simulink model "Project2"  (R2015a)
settings: Solver=ode45  StartTime=0.0  StopTime=10000  RelTol=1e-3
PreLoadFcn:
  | Init
InitFcn:
  | Init
values from neighbouring files (symbols this model uses):
  a = 5    [Init.m]
  b = 10    [Init.m]
  PACCPrecision = 32    [Init.m]
  seed = [1,2,3,4,5,6]    [Init.m]
undefined symbols (not defined in the file or in its folder): c
libraries: xbsIndex_r4 x91, xrbsComm_r4 x1
(part 2 of 2)

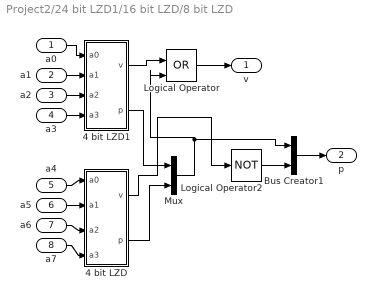
== system Project2/24 bit LZD1/16 bit LZD/8 bit LZD ==
  a0 : Inport
  a1 : Inport  Port=2
  a2 : Inport  Port=3
  a3 : Inport  Port=4
  a4 : Inport  Port=5
  a5 : Inport  Port=6
  a6 : Inport  Port=7
  a7 : Inport  Port=8
  4 bit LZD : Subsystem
  4 bit LZD1 : Subsystem
  Bus Creator1 : BusCreator  Inputs=2
  Logical Operator : Logic  Operator=OR  IconShape=distinctive  AllPortsSameDT=off  OutDataTypeStr=boolean
  Logical Operator2 : Logic  Operator=NOT  IconShape=distinctive  AllPortsSameDT=off  OutDataTypeStr=boolean
  Mux : Mux  Inputs=2
  v : Outport
  p : Outport  Port=2
  wires:
  a2/1 -> 4 bit LZD1/3(a2)
  a6/1 -> 4 bit LZD/3(a2)
  a7/1 -> 4 bit LZD/4(a3)
  a3/1 -> 4 bit LZD1/4(a3)
  a0/1 -> 4 bit LZD1/1(a0)
  a1/1 -> 4 bit LZD1/2(a1)
  a5/1 -> 4 bit LZD/2(a1)
  a4/1 -> 4 bit LZD/1(a0)
  Logical Operator/1 -> v/1
  Logical Operator2/1 -> Bus Creator1/2
  4 bit LZD1/1(v) -> Logical Operator/1
  Mux/1 -> Logical Operator/2, Bus Creator1/1
  4 bit LZD/2(p) -> Mux/2
  Bus Creator1/1 -> p/1
  4 bit LZD/1(v) -> Logical Operator2/1
  4 bit LZD1/2(p) -> Mux/1

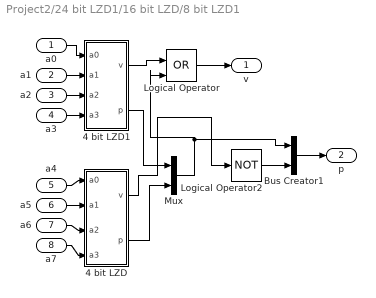
== system Project2/24 bit LZD1/16 bit LZD/8 bit LZD1 ==
  a0 : Inport
  a1 : Inport  Port=2
  a2 : Inport  Port=3
  a3 : Inport  Port=4
  a4 : Inport  Port=5
  a5 : Inport  Port=6
  a6 : Inport  Port=7
  a7 : Inport  Port=8
  4 bit LZD : Subsystem
  4 bit LZD1 : Subsystem
  Bus Creator1 : BusCreator  Inputs=2
  Logical Operator : Logic  Operator=OR  IconShape=distinctive  AllPortsSameDT=off  OutDataTypeStr=boolean
  Logical Operator2 : Logic  Operator=NOT  IconShape=distinctive  AllPortsSameDT=off  OutDataTypeStr=boolean
  Mux : Mux  Inputs=2
  v : Outport
  p : Outport  Port=2
  wires:
  a2/1 -> 4 bit LZD1/3(a2)
  a6/1 -> 4 bit LZD/3(a2)
  a7/1 -> 4 bit LZD/4(a3)
  a3/1 -> 4 bit LZD1/4(a3)
  a0/1 -> 4 bit LZD1/1(a0)
  a1/1 -> 4 bit LZD1/2(a1)
  a5/1 -> 4 bit LZD/2(a1)
  a4/1 -> 4 bit LZD/1(a0)
  Logical Operator/1 -> v/1
  Logical Operator2/1 -> Bus Creator1/2
  4 bit LZD1/1(v) -> Logical Operator/1
  Mux/1 -> Logical Operator/2, Bus Creator1/1
  4 bit LZD/2(p) -> Mux/2
  Bus Creator1/1 -> p/1
  4 bit LZD/1(v) -> Logical Operator2/1
  4 bit LZD1/2(p) -> Mux/1

== system Project2/24 bit LZD1/8 bit LZD/4 bit LZD ==
  a0 : Inport
  a1 : Inport  Port=2
  a2 : Inport  Port=3
  a3 : Inport  Port=4
  2 bit LZD : Subsystem
  2 bit LZD1 : Subsystem
  Bus Creator1 : BusCreator  Inputs=2
  Logical Operator : Logic  Operator=OR  IconShape=distinctive  AllPortsSameDT=off  OutDataTypeStr=boolean
  Logical Operator2 : Logic  Operator=NOT  IconShape=distinctive  AllPortsSameDT=off  OutDataTypeStr=boolean
  Mux : Mux  Inputs=2
  v : Outport
  p : Outport  Port=2
  wires:
  2 bit LZD/1(v) -> Logical Operator2/1
  2 bit LZD1/2(p) -> Mux/1
  2 bit LZD/2(p) -> Mux/2
  Bus Creator1/1 -> p/1
  a0/1 -> 2 bit LZD1/1(a0)
  a2/1 -> 2 bit LZD/1(a0)
  a1/1 -> 2 bit LZD1/2(a1)
  a3/1 -> 2 bit LZD/2(a1)
  Logical Operator/1 -> v/1
  2 bit LZD1/1(v) -> Logical Operator/1
  Logical Operator2/1 -> Bus Creator1/2
  Mux/1 -> Logical Operator/2, Bus Creator1/1

== system Project2/24 bit LZD1/8 bit LZD/4 bit LZD1 ==
  a0 : Inport
  a1 : Inport  Port=2
  a2 : Inport  Port=3
  a3 : Inport  Port=4
  2 bit LZD : Subsystem
  2 bit LZD1 : Subsystem
  Bus Creator1 : BusCreator  Inputs=2
  Logical Operator : Logic  Operator=OR  IconShape=distinctive  AllPortsSameDT=off  OutDataTypeStr=boolean
  Logical Operator2 : Logic  Operator=NOT  IconShape=distinctive  AllPortsSameDT=off  OutDataTypeStr=boolean
  Mux : Mux  Inputs=2
  v : Outport
  p : Outport  Port=2
  wires:
  2 bit LZD/1(v) -> Logical Operator2/1
  2 bit LZD1/2(p) -> Mux/1
  2 bit LZD/2(p) -> Mux/2
  Bus Creator1/1 -> p/1
  a0/1 -> 2 bit LZD1/1(a0)
  a2/1 -> 2 bit LZD/1(a0)
  a1/1 -> 2 bit LZD1/2(a1)
  a3/1 -> 2 bit LZD/2(a1)
  Logical Operator/1 -> v/1
  2 bit LZD1/1(v) -> Logical Operator/1
  Logical Operator2/1 -> Bus Creator1/2
  Mux/1 -> Logical Operator/2, Bus Creator1/1

== system Project2/24 bit LZD/16 bit LZD/8 bit LZD/4 bit LZD ==
  a0 : Inport
  a1 : Inport  Port=2
  a2 : Inport  Port=3
  a3 : Inport  Port=4
  2 bit LZD : Subsystem
  2 bit LZD1 : Subsystem
  Bus Creator1 : BusCreator  Inputs=2
  Logical Operator : Logic  Operator=OR  IconShape=distinctive  AllPortsSameDT=off  OutDataTypeStr=boolean
  Logical Operator2 : Logic  Operator=NOT  IconShape=distinctive  AllPortsSameDT=off  OutDataTypeStr=boolean
  Mux : Mux  Inputs=2
  v : Outport
  p : Outport  Port=2
  wires:
  2 bit LZD/1(v) -> Logical Operator2/1
  2 bit LZD1/2(p) -> Mux/1
  2 bit LZD/2(p) -> Mux/2
  Bus Creator1/1 -> p/1
  a0/1 -> 2 bit LZD1/1(a0)
  a2/1 -> 2 bit LZD/1(a0)
  a1/1 -> 2 bit LZD1/2(a1)
  a3/1 -> 2 bit LZD/2(a1)
  Logical Operator/1 -> v/1
  2 bit LZD1/1(v) -> Logical Operator/1
  Logical Operator2/1 -> Bus Creator1/2
  Mux/1 -> Logical Operator/2, Bus Creator1/1

== system Project2/24 bit LZD/16 bit LZD/8 bit LZD/4 bit LZD1 ==
  a0 : Inport
  a1 : Inport  Port=2
  a2 : Inport  Port=3
  a3 : Inport  Port=4
  2 bit LZD : Subsystem
  2 bit LZD1 : Subsystem
  Bus Creator1 : BusCreator  Inputs=2
  Logical Operator : Logic  Operator=OR  IconShape=distinctive  AllPortsSameDT=off  OutDataTypeStr=boolean
  Logical Operator2 : Logic  Operator=NOT  IconShape=distinctive  AllPortsSameDT=off  OutDataTypeStr=boolean
  Mux : Mux  Inputs=2
  v : Outport
  p : Outport  Port=2
  wires:
  2 bit LZD/1(v) -> Logical Operator2/1
  2 bit LZD1/2(p) -> Mux/1
  2 bit LZD/2(p) -> Mux/2
  Bus Creator1/1 -> p/1
  a0/1 -> 2 bit LZD1/1(a0)
  a2/1 -> 2 bit LZD/1(a0)
  a1/1 -> 2 bit LZD1/2(a1)
  a3/1 -> 2 bit LZD/2(a1)
  Logical Operator/1 -> v/1
  2 bit LZD1/1(v) -> Logical Operator/1
  Logical Operator2/1 -> Bus Creator1/2
  Mux/1 -> Logical Operator/2, Bus Creator1/1

== system Project2/24 bit LZD/16 bit LZD/8 bit LZD1/4 bit LZD ==
  a0 : Inport
  a1 : Inport  Port=2
  a2 : Inport  Port=3
  a3 : Inport  Port=4
  2 bit LZD : Subsystem
  2 bit LZD1 : Subsystem
  Bus Creator1 : BusCreator  Inputs=2
  Logical Operator : Logic  Operator=OR  IconShape=distinctive  AllPortsSameDT=off  OutDataTypeStr=boolean
  Logical Operator2 : Logic  Operator=NOT  IconShape=distinctive  AllPortsSameDT=off  OutDataTypeStr=boolean
  Mux : Mux  Inputs=2
  v : Outport
  p : Outport  Port=2
  wires:
  2 bit LZD/1(v) -> Logical Operator2/1
  2 bit LZD1/2(p) -> Mux/1
  2 bit LZD/2(p) -> Mux/2
  Bus Creator1/1 -> p/1
  a0/1 -> 2 bit LZD1/1(a0)
  a2/1 -> 2 bit LZD/1(a0)
  a1/1 -> 2 bit LZD1/2(a1)
  a3/1 -> 2 bit LZD/2(a1)
  Logical Operator/1 -> v/1
  2 bit LZD1/1(v) -> Logical Operator/1
  Logical Operator2/1 -> Bus Creator1/2
  Mux/1 -> Logical Operator/2, Bus Creator1/1

== system Project2/24 bit LZD/16 bit LZD/8 bit LZD1/4 bit LZD1 ==
  a0 : Inport
  a1 : Inport  Port=2
  a2 : Inport  Port=3
  a3 : Inport  Port=4
  2 bit LZD : Subsystem
  2 bit LZD1 : Subsystem
  Bus Creator1 : BusCreator  Inputs=2
  Logical Operator : Logic  Operator=OR  IconShape=distinctive  AllPortsSameDT=off  OutDataTypeStr=boolean
  Logical Operator2 : Logic  Operator=NOT  IconShape=distinctive  AllPortsSameDT=off  OutDataTypeStr=boolean
  Mux : Mux  Inputs=2
  v : Outport
  p : Outport  Port=2
  wires:
  2 bit LZD/1(v) -> Logical Operator2/1
  2 bit LZD1/2(p) -> Mux/1
  2 bit LZD/2(p) -> Mux/2
  Bus Creator1/1 -> p/1
  a0/1 -> 2 bit LZD1/1(a0)
  a2/1 -> 2 bit LZD/1(a0)
  a1/1 -> 2 bit LZD1/2(a1)
  a3/1 -> 2 bit LZD/2(a1)
  Logical Operator/1 -> v/1
  2 bit LZD1/1(v) -> Logical Operator/1
  Logical Operator2/1 -> Bus Creator1/2
  Mux/1 -> Logical Operator/2, Bus Creator1/1

== system Project2/24 bit LZD/8 bit LZD/4 bit LZD/2 bit LZD ==
  a0 : Inport
  a1 : Inport  Port=2
  Logical Operator : Logic  Operator=OR  IconShape=distinctive  AllPortsSameDT=off  OutDataTypeStr=boolean
  Logical Operator1 : Logic  IconShape=distinctive  AllPortsSameDT=off  OutDataTypeStr=boolean
  Logical Operator2 : Logic  Operator=NOT  IconShape=distinctive  AllPortsSameDT=off  OutDataTypeStr=boolean
  v : Outport
  p : Outport  Port=2
  wires:
  Logical Operator/1 -> v/1
  Logical Operator2/1 -> Logical Operator1/2
  a0/1 -> Logical Operator1/1, Logical Operator/1
  Logical Operator1/1 -> p/1
  a1/1 -> Logical Operator/2, Logical Operator2/1

== system Project2/24 bit LZD/8 bit LZD/4 bit LZD/2 bit LZD1 ==
  a0 : Inport
  a1 : Inport  Port=2
  Logical Operator : Logic  Operator=OR  IconShape=distinctive  AllPortsSameDT=off  OutDataTypeStr=boolean
  Logical Operator1 : Logic  IconShape=distinctive  AllPortsSameDT=off  OutDataTypeStr=boolean
  Logical Operator2 : Logic  Operator=NOT  IconShape=distinctive  AllPortsSameDT=off  OutDataTypeStr=boolean
  v : Outport
  p : Outport  Port=2
  wires:
  Logical Operator/1 -> v/1
  Logical Operator2/1 -> Logical Operator1/2
  a0/1 -> Logical Operator1/1, Logical Operator/1
  Logical Operator1/1 -> p/1
  a1/1 -> Logical Operator/2, Logical Operator2/1

== system Project2/24 bit LZD/8 bit LZD/4 bit LZD1/2 bit LZD ==
  a0 : Inport
  a1 : Inport  Port=2
  Logical Operator : Logic  Operator=OR  IconShape=distinctive  AllPortsSameDT=off  OutDataTypeStr=boolean
  Logical Operator1 : Logic  IconShape=distinctive  AllPortsSameDT=off  OutDataTypeStr=boolean
  Logical Operator2 : Logic  Operator=NOT  IconShape=distinctive  AllPortsSameDT=off  OutDataTypeStr=boolean
  v : Outport
  p : Outport  Port=2
  wires:
  Logical Operator/1 -> v/1
  Logical Operator2/1 -> Logical Operator1/2
  a0/1 -> Logical Operator1/1, Logical Operator/1
  Logical Operator1/1 -> p/1
  a1/1 -> Logical Operator/2, Logical Operator2/1

== system Project2/24 bit LZD/8 bit LZD/4 bit LZD1/2 bit LZD1 ==
  a0 : Inport
  a1 : Inport  Port=2
  Logical Operator : Logic  Operator=OR  IconShape=distinctive  AllPortsSameDT=off  OutDataTypeStr=boolean
  Logical Operator1 : Logic  IconShape=distinctive  AllPortsSameDT=off  OutDataTypeStr=boolean
  Logical Operator2 : Logic  Operator=NOT  IconShape=distinctive  AllPortsSameDT=off  OutDataTypeStr=boolean
  v : Outport
  p : Outport  Port=2
  wires:
  Logical Operator/1 -> v/1
  Logical Operator2/1 -> Logical Operator1/2
  a0/1 -> Logical Operator1/1, Logical Operator/1
  Logical Operator1/1 -> p/1
  a1/1 -> Logical Operator/2, Logical Operator2/1

== system Project2/24 bit LZD1/16 bit LZD/8 bit LZD/4 bit LZD ==
  a0 : Inport
  a1 : Inport  Port=2
  a2 : Inport  Port=3
  a3 : Inport  Port=4
  2 bit LZD : Subsystem
  2 bit LZD1 : Subsystem
  Bus Creator1 : BusCreator  Inputs=2
  Logical Operator : Logic  Operator=OR  IconShape=distinctive  AllPortsSameDT=off  OutDataTypeStr=boolean
  Logical Operator2 : Logic  Operator=NOT  IconShape=distinctive  AllPortsSameDT=off  OutDataTypeStr=boolean
  Mux : Mux  Inputs=2
  v : Outport
  p : Outport  Port=2
  wires:
  2 bit LZD/1(v) -> Logical Operator2/1
  2 bit LZD1/2(p) -> Mux/1
  2 bit LZD/2(p) -> Mux/2
  Bus Creator1/1 -> p/1
  a0/1 -> 2 bit LZD1/1(a0)
  a2/1 -> 2 bit LZD/1(a0)
  a1/1 -> 2 bit LZD1/2(a1)
  a3/1 -> 2 bit LZD/2(a1)
  Logical Operator/1 -> v/1
  2 bit LZD1/1(v) -> Logical Operator/1
  Logical Operator2/1 -> Bus Creator1/2
  Mux/1 -> Logical Operator/2, Bus Creator1/1

== system Project2/24 bit LZD1/16 bit LZD/8 bit LZD/4 bit LZD1 ==
  a0 : Inport
  a1 : Inport  Port=2
  a2 : Inport  Port=3
  a3 : Inport  Port=4
  2 bit LZD : Subsystem
  2 bit LZD1 : Subsystem
  Bus Creator1 : BusCreator  Inputs=2
  Logical Operator : Logic  Operator=OR  IconShape=distinctive  AllPortsSameDT=off  OutDataTypeStr=boolean
  Logical Operator2 : Logic  Operator=NOT  IconShape=distinctive  AllPortsSameDT=off  OutDataTypeStr=boolean
  Mux : Mux  Inputs=2
  v : Outport
  p : Outport  Port=2
  wires:
  2 bit LZD/1(v) -> Logical Operator2/1
  2 bit LZD1/2(p) -> Mux/1
  2 bit LZD/2(p) -> Mux/2
  Bus Creator1/1 -> p/1
  a0/1 -> 2 bit LZD1/1(a0)
  a2/1 -> 2 bit LZD/1(a0)
  a1/1 -> 2 bit LZD1/2(a1)
  a3/1 -> 2 bit LZD/2(a1)
  Logical Operator/1 -> v/1
  2 bit LZD1/1(v) -> Logical Operator/1
  Logical Operator2/1 -> Bus Creator1/2
  Mux/1 -> Logical Operator/2, Bus Creator1/1

== system Project2/24 bit LZD1/16 bit LZD/8 bit LZD1/4 bit LZD ==
  a0 : Inport
  a1 : Inport  Port=2
  a2 : Inport  Port=3
  a3 : Inport  Port=4
  2 bit LZD : Subsystem
  2 bit LZD1 : Subsystem
  Bus Creator1 : BusCreator  Inputs=2
  Logical Operator : Logic  Operator=OR  IconShape=distinctive  AllPortsSameDT=off  OutDataTypeStr=boolean
  Logical Operator2 : Logic  Operator=NOT  IconShape=distinctive  AllPortsSameDT=off  OutDataTypeStr=boolean
  Mux : Mux  Inputs=2
  v : Outport
  p : Outport  Port=2
  wires:
  2 bit LZD/1(v) -> Logical Operator2/1
  2 bit LZD1/2(p) -> Mux/1
  2 bit LZD/2(p) -> Mux/2
  Bus Creator1/1 -> p/1
  a0/1 -> 2 bit LZD1/1(a0)
  a2/1 -> 2 bit LZD/1(a0)
  a1/1 -> 2 bit LZD1/2(a1)
  a3/1 -> 2 bit LZD/2(a1)
  Logical Operator/1 -> v/1
  2 bit LZD1/1(v) -> Logical Operator/1
  Logical Operator2/1 -> Bus Creator1/2
  Mux/1 -> Logical Operator/2, Bus Creator1/1

== system Project2/24 bit LZD1/16 bit LZD/8 bit LZD1/4 bit LZD1 ==
  a0 : Inport
  a1 : Inport  Port=2
  a2 : Inport  Port=3
  a3 : Inport  Port=4
  2 bit LZD : Subsystem
  2 bit LZD1 : Subsystem
  Bus Creator1 : BusCreator  Inputs=2
  Logical Operator : Logic  Operator=OR  IconShape=distinctive  AllPortsSameDT=off  OutDataTypeStr=boolean
  Logical Operator2 : Logic  Operator=NOT  IconShape=distinctive  AllPortsSameDT=off  OutDataTypeStr=boolean
  Mux : Mux  Inputs=2
  v : Outport
  p : Outport  Port=2
  wires:
  2 bit LZD/1(v) -> Logical Operator2/1
  2 bit LZD1/2(p) -> Mux/1
  2 bit LZD/2(p) -> Mux/2
  Bus Creator1/1 -> p/1
  a0/1 -> 2 bit LZD1/1(a0)
  a2/1 -> 2 bit LZD/1(a0)
  a1/1 -> 2 bit LZD1/2(a1)
  a3/1 -> 2 bit LZD/2(a1)
  Logical Operator/1 -> v/1
  2 bit LZD1/1(v) -> Logical Operator/1
  Logical Operator2/1 -> Bus Creator1/2
  Mux/1 -> Logical Operator/2, Bus Creator1/1

== system Project2/24 bit LZD1/8 bit LZD/4 bit LZD/2 bit LZD ==
  a0 : Inport
  a1 : Inport  Port=2
  Logical Operator : Logic  Operator=OR  IconShape=distinctive  AllPortsSameDT=off  OutDataTypeStr=boolean
  Logical Operator1 : Logic  IconShape=distinctive  AllPortsSameDT=off  OutDataTypeStr=boolean
  Logical Operator2 : Logic  Operator=NOT  IconShape=distinctive  AllPortsSameDT=off  OutDataTypeStr=boolean
  v : Outport
  p : Outport  Port=2
  wires:
  Logical Operator/1 -> v/1
  Logical Operator2/1 -> Logical Operator1/2
  a0/1 -> Logical Operator1/1, Logical Operator/1
  Logical Operator1/1 -> p/1
  a1/1 -> Logical Operator/2, Logical Operator2/1

== system Project2/24 bit LZD1/8 bit LZD/4 bit LZD/2 bit LZD1 ==
  a0 : Inport
  a1 : Inport  Port=2
  Logical Operator : Logic  Operator=OR  IconShape=distinctive  AllPortsSameDT=off  OutDataTypeStr=boolean
  Logical Operator1 : Logic  IconShape=distinctive  AllPortsSameDT=off  OutDataTypeStr=boolean
  Logical Operator2 : Logic  Operator=NOT  IconShape=distinctive  AllPortsSameDT=off  OutDataTypeStr=boolean
  v : Outport
  p : Outport  Port=2
  wires:
  Logical Operator/1 -> v/1
  Logical Operator2/1 -> Logical Operator1/2
  a0/1 -> Logical Operator1/1, Logical Operator/1
  Logical Operator1/1 -> p/1
  a1/1 -> Logical Operator/2, Logical Operator2/1

== system Project2/24 bit LZD1/8 bit LZD/4 bit LZD1/2 bit LZD ==
  a0 : Inport
  a1 : Inport  Port=2
  Logical Operator : Logic  Operator=OR  IconShape=distinctive  AllPortsSameDT=off  OutDataTypeStr=boolean
  Logical Operator1 : Logic  IconShape=distinctive  AllPortsSameDT=off  OutDataTypeStr=boolean
  Logical Operator2 : Logic  Operator=NOT  IconShape=distinctive  AllPortsSameDT=off  OutDataTypeStr=boolean
  v : Outport
  p : Outport  Port=2
  wires:
  Logical Operator/1 -> v/1
  Logical Operator2/1 -> Logical Operator1/2
  a0/1 -> Logical Operator1/1, Logical Operator/1
  Logical Operator1/1 -> p/1
  a1/1 -> Logical Operator/2, Logical Operator2/1

== system Project2/24 bit LZD1/8 bit LZD/4 bit LZD1/2 bit LZD1 ==
  a0 : Inport
  a1 : Inport  Port=2
  Logical Operator : Logic  Operator=OR  IconShape=distinctive  AllPortsSameDT=off  OutDataTypeStr=boolean
  Logical Operator1 : Logic  IconShape=distinctive  AllPortsSameDT=off  OutDataTypeStr=boolean
  Logical Operator2 : Logic  Operator=NOT  IconShape=distinctive  AllPortsSameDT=off  OutDataTypeStr=boolean
  v : Outport
  p : Outport  Port=2
  wires:
  Logical Operator/1 -> v/1
  Logical Operator2/1 -> Logical Operator1/2
  a0/1 -> Logical Operator1/1, Logical Operator/1
  Logical Operator1/1 -> p/1
  a1/1 -> Logical Operator/2, Logical Operator2/1

== system Project2/24 bit LZD/16 bit LZD/8 bit LZD/4 bit LZD/2 bit LZD ==
  a0 : Inport
  a1 : Inport  Port=2
  Logical Operator : Logic  Operator=OR  IconShape=distinctive  AllPortsSameDT=off  OutDataTypeStr=boolean
  Logical Operator1 : Logic  IconShape=distinctive  AllPortsSameDT=off  OutDataTypeStr=boolean
  Logical Operator2 : Logic  Operator=NOT  IconShape=distinctive  AllPortsSameDT=off  OutDataTypeStr=boolean
  v : Outport
  p : Outport  Port=2
  wires:
  Logical Operator/1 -> v/1
  Logical Operator2/1 -> Logical Operator1/2
  a0/1 -> Logical Operator1/1, Logical Operator/1
  Logical Operator1/1 -> p/1
  a1/1 -> Logical Operator/2, Logical Operator2/1

== system Project2/24 bit LZD/16 bit LZD/8 bit LZD/4 bit LZD/2 bit LZD1 ==
  a0 : Inport
  a1 : Inport  Port=2
  Logical Operator : Logic  Operator=OR  IconShape=distinctive  AllPortsSameDT=off  OutDataTypeStr=boolean
  Logical Operator1 : Logic  IconShape=distinctive  AllPortsSameDT=off  OutDataTypeStr=boolean
  Logical Operator2 : Logic  Operator=NOT  IconShape=distinctive  AllPortsSameDT=off  OutDataTypeStr=boolean
  v : Outport
  p : Outport  Port=2
  wires:
  Logical Operator/1 -> v/1
  Logical Operator2/1 -> Logical Operator1/2
  a0/1 -> Logical Operator1/1, Logical Operator/1
  Logical Operator1/1 -> p/1
  a1/1 -> Logical Operator/2, Logical Operator2/1

== system Project2/24 bit LZD/16 bit LZD/8 bit LZD/4 bit LZD1/2 bit LZD ==
  a0 : Inport
  a1 : Inport  Port=2
  Logical Operator : Logic  Operator=OR  IconShape=distinctive  AllPortsSameDT=off  OutDataTypeStr=boolean
  Logical Operator1 : Logic  IconShape=distinctive  AllPortsSameDT=off  OutDataTypeStr=boolean
  Logical Operator2 : Logic  Operator=NOT  IconShape=distinctive  AllPortsSameDT=off  OutDataTypeStr=boolean
  v : Outport
  p : Outport  Port=2
  wires:
  Logical Operator/1 -> v/1
  Logical Operator2/1 -> Logical Operator1/2
  a0/1 -> Logical Operator1/1, Logical Operator/1
  Logical Operator1/1 -> p/1
  a1/1 -> Logical Operator/2, Logical Operator2/1

== system Project2/24 bit LZD/16 bit LZD/8 bit LZD/4 bit LZD1/2 bit LZD1 ==
  a0 : Inport
  a1 : Inport  Port=2
  Logical Operator : Logic  Operator=OR  IconShape=distinctive  AllPortsSameDT=off  OutDataTypeStr=boolean
  Logical Operator1 : Logic  IconShape=distinctive  AllPortsSameDT=off  OutDataTypeStr=boolean
  Logical Operator2 : Logic  Operator=NOT  IconShape=distinctive  AllPortsSameDT=off  OutDataTypeStr=boolean
  v : Outport
  p : Outport  Port=2
  wires:
  Logical Operator/1 -> v/1
  Logical Operator2/1 -> Logical Operator1/2
  a0/1 -> Logical Operator1/1, Logical Operator/1
  Logical Operator1/1 -> p/1
  a1/1 -> Logical Operator/2, Logical Operator2/1

== system Project2/24 bit LZD/16 bit LZD/8 bit LZD1/4 bit LZD/2 bit LZD ==
  a0 : Inport
  a1 : Inport  Port=2
  Logical Operator : Logic  Operator=OR  IconShape=distinctive  AllPortsSameDT=off  OutDataTypeStr=boolean
  Logical Operator1 : Logic  IconShape=distinctive  AllPortsSameDT=off  OutDataTypeStr=boolean
  Logical Operator2 : Logic  Operator=NOT  IconShape=distinctive  AllPortsSameDT=off  OutDataTypeStr=boolean
  v : Outport
  p : Outport  Port=2
  wires:
  Logical Operator/1 -> v/1
  Logical Operator2/1 -> Logical Operator1/2
  a0/1 -> Logical Operator1/1, Logical Operator/1
  Logical Operator1/1 -> p/1
  a1/1 -> Logical Operator/2, Logical Operator2/1

== system Project2/24 bit LZD/16 bit LZD/8 bit LZD1/4 bit LZD/2 bit LZD1 ==
  a0 : Inport
  a1 : Inport  Port=2
  Logical Operator : Logic  Operator=OR  IconShape=distinctive  AllPortsSameDT=off  OutDataTypeStr=boolean
  Logical Operator1 : Logic  IconShape=distinctive  AllPortsSameDT=off  OutDataTypeStr=boolean
  Logical Operator2 : Logic  Operator=NOT  IconShape=distinctive  AllPortsSameDT=off  OutDataTypeStr=boolean
  v : Outport
  p : Outport  Port=2
  wires:
  Logical Operator/1 -> v/1
  Logical Operator2/1 -> Logical Operator1/2
  a0/1 -> Logical Operator1/1, Logical Operator/1
  Logical Operator1/1 -> p/1
  a1/1 -> Logical Operator/2, Logical Operator2/1

== system Project2/24 bit LZD/16 bit LZD/8 bit LZD1/4 bit LZD1/2 bit LZD ==
  a0 : Inport
  a1 : Inport  Port=2
  Logical Operator : Logic  Operator=OR  IconShape=distinctive  AllPortsSameDT=off  OutDataTypeStr=boolean
  Logical Operator1 : Logic  IconShape=distinctive  AllPortsSameDT=off  OutDataTypeStr=boolean
  Logical Operator2 : Logic  Operator=NOT  IconShape=distinctive  AllPortsSameDT=off  OutDataTypeStr=boolean
  v : Outport
  p : Outport  Port=2
  wires:
  Logical Operator/1 -> v/1
  Logical Operator2/1 -> Logical Operator1/2
  a0/1 -> Logical Operator1/1, Logical Operator/1
  Logical Operator1/1 -> p/1
  a1/1 -> Logical Operator/2, Logical Operator2/1

== system Project2/24 bit LZD/16 bit LZD/8 bit LZD1/4 bit LZD1/2 bit LZD1 ==
  a0 : Inport
  a1 : Inport  Port=2
  Logical Operator : Logic  Operator=OR  IconShape=distinctive  AllPortsSameDT=off  OutDataTypeStr=boolean
  Logical Operator1 : Logic  IconShape=distinctive  AllPortsSameDT=off  OutDataTypeStr=boolean
  Logical Operator2 : Logic  Operator=NOT  IconShape=distinctive  AllPortsSameDT=off  OutDataTypeStr=boolean
  v : Outport
  p : Outport  Port=2
  wires:
  Logical Operator/1 -> v/1
  Logical Operator2/1 -> Logical Operator1/2
  a0/1 -> Logical Operator1/1, Logical Operator/1
  Logical Operator1/1 -> p/1
  a1/1 -> Logical Operator/2, Logical Operator2/1

== system Project2/24 bit LZD1/16 bit LZD/8 bit LZD/4 bit LZD/2 bit LZD ==
  a0 : Inport
  a1 : Inport  Port=2
  Logical Operator : Logic  Operator=OR  IconShape=distinctive  AllPortsSameDT=off  OutDataTypeStr=boolean
  Logical Operator1 : Logic  IconShape=distinctive  AllPortsSameDT=off  OutDataTypeStr=boolean
  Logical Operator2 : Logic  Operator=NOT  IconShape=distinctive  AllPortsSameDT=off  OutDataTypeStr=boolean
  v : Outport
  p : Outport  Port=2
  wires:
  Logical Operator/1 -> v/1
  Logical Operator2/1 -> Logical Operator1/2
  a0/1 -> Logical Operator1/1, Logical Operator/1
  Logical Operator1/1 -> p/1
  a1/1 -> Logical Operator/2, Logical Operator2/1

== system Project2/24 bit LZD1/16 bit LZD/8 bit LZD/4 bit LZD/2 bit LZD1 ==
  a0 : Inport
  a1 : Inport  Port=2
  Logical Operator : Logic  Operator=OR  IconShape=distinctive  AllPortsSameDT=off  OutDataTypeStr=boolean
  Logical Operator1 : Logic  IconShape=distinctive  AllPortsSameDT=off  OutDataTypeStr=boolean
  Logical Operator2 : Logic  Operator=NOT  IconShape=distinctive  AllPortsSameDT=off  OutDataTypeStr=boolean
  v : Outport
  p : Outport  Port=2
  wires:
  Logical Operator/1 -> v/1
  Logical Operator2/1 -> Logical Operator1/2
  a0/1 -> Logical Operator1/1, Logical Operator/1
  Logical Operator1/1 -> p/1
  a1/1 -> Logical Operator/2, Logical Operator2/1

== system Project2/24 bit LZD1/16 bit LZD/8 bit LZD/4 bit LZD1/2 bit LZD ==
  a0 : Inport
  a1 : Inport  Port=2
  Logical Operator : Logic  Operator=OR  IconShape=distinctive  AllPortsSameDT=off  OutDataTypeStr=boolean
  Logical Operator1 : Logic  IconShape=distinctive  AllPortsSameDT=off  OutDataTypeStr=boolean
  Logical Operator2 : Logic  Operator=NOT  IconShape=distinctive  AllPortsSameDT=off  OutDataTypeStr=boolean
  v : Outport
  p : Outport  Port=2
  wires:
  Logical Operator/1 -> v/1
  Logical Operator2/1 -> Logical Operator1/2
  a0/1 -> Logical Operator1/1, Logical Operator/1
  Logical Operator1/1 -> p/1
  a1/1 -> Logical Operator/2, Logical Operator2/1

== system Project2/24 bit LZD1/16 bit LZD/8 bit LZD/4 bit LZD1/2 bit LZD1 ==
  a0 : Inport
  a1 : Inport  Port=2
  Logical Operator : Logic  Operator=OR  IconShape=distinctive  AllPortsSameDT=off  OutDataTypeStr=boolean
  Logical Operator1 : Logic  IconShape=distinctive  AllPortsSameDT=off  OutDataTypeStr=boolean
  Logical Operator2 : Logic  Operator=NOT  IconShape=distinctive  AllPortsSameDT=off  OutDataTypeStr=boolean
  v : Outport
  p : Outport  Port=2
  wires:
  Logical Operator/1 -> v/1
  Logical Operator2/1 -> Logical Operator1/2
  a0/1 -> Logical Operator1/1, Logical Operator/1
  Logical Operator1/1 -> p/1
  a1/1 -> Logical Operator/2, Logical Operator2/1

== system Project2/24 bit LZD1/16 bit LZD/8 bit LZD1/4 bit LZD/2 bit LZD ==
  a0 : Inport
  a1 : Inport  Port=2
  Logical Operator : Logic  Operator=OR  IconShape=distinctive  AllPortsSameDT=off  OutDataTypeStr=boolean
  Logical Operator1 : Logic  IconShape=distinctive  AllPortsSameDT=off  OutDataTypeStr=boolean
  Logical Operator2 : Logic  Operator=NOT  IconShape=distinctive  AllPortsSameDT=off  OutDataTypeStr=boolean
  v : Outport
  p : Outport  Port=2
  wires:
  Logical Operator/1 -> v/1
  Logical Operator2/1 -> Logical Operator1/2
  a0/1 -> Logical Operator1/1, Logical Operator/1
  Logical Operator1/1 -> p/1
  a1/1 -> Logical Operator/2, Logical Operator2/1

== system Project2/24 bit LZD1/16 bit LZD/8 bit LZD1/4 bit LZD/2 bit LZD1 ==
  a0 : Inport
  a1 : Inport  Port=2
  Logical Operator : Logic  Operator=OR  IconShape=distinctive  AllPortsSameDT=off  OutDataTypeStr=boolean
  Logical Operator1 : Logic  IconShape=distinctive  AllPortsSameDT=off  OutDataTypeStr=boolean
  Logical Operator2 : Logic  Operator=NOT  IconShape=distinctive  AllPortsSameDT=off  OutDataTypeStr=boolean
  v : Outport
  p : Outport  Port=2
  wires:
  Logical Operator/1 -> v/1
  Logical Operator2/1 -> Logical Operator1/2
  a0/1 -> Logical Operator1/1, Logical Operator/1
  Logical Operator1/1 -> p/1
  a1/1 -> Logical Operator/2, Logical Operator2/1

== system Project2/24 bit LZD1/16 bit LZD/8 bit LZD1/4 bit LZD1/2 bit LZD ==
  a0 : Inport
  a1 : Inport  Port=2
  Logical Operator : Logic  Operator=OR  IconShape=distinctive  AllPortsSameDT=off  OutDataTypeStr=boolean
  Logical Operator1 : Logic  IconShape=distinctive  AllPortsSameDT=off  OutDataTypeStr=boolean
  Logical Operator2 : Logic  Operator=NOT  IconShape=distinctive  AllPortsSameDT=off  OutDataTypeStr=boolean
  v : Outport
  p : Outport  Port=2
  wires:
  Logical Operator/1 -> v/1
  Logical Operator2/1 -> Logical Operator1/2
  a0/1 -> Logical Operator1/1, Logical Operator/1
  Logical Operator1/1 -> p/1
  a1/1 -> Logical Operator/2, Logical Operator2/1

== system Project2/24 bit LZD1/16 bit LZD/8 bit LZD1/4 bit LZD1/2 bit LZD1 ==
  a0 : Inport
  a1 : Inport  Port=2
  Logical Operator : Logic  Operator=OR  IconShape=distinctive  AllPortsSameDT=off  OutDataTypeStr=boolean
  Logical Operator1 : Logic  IconShape=distinctive  AllPortsSameDT=off  OutDataTypeStr=boolean
  Logical Operator2 : Logic  Operator=NOT  IconShape=distinctive  AllPortsSameDT=off  OutDataTypeStr=boolean
  v : Outport
  p : Outport  Port=2
  wires:
  Logical Operator/1 -> v/1
  Logical Operator2/1 -> Logical Operator1/2
  a0/1 -> Logical Operator1/1, Logical Operator/1
  Logical Operator1/1 -> p/1
  a1/1 -> Logical Operator/2, Logical Operator2/1
